simulink model "Vehicle_suspension"  (R2020b)
settings: Solver=VariableStepAuto  StartTime=0.0  StopTime=10.0  RelTol=1e-3
values from neighbouring files (symbols this model uses):
  Iyy = 2100.0    [data_dictionary.sldd]
  Mb = 1200.0    [data_dictionary.sldd]
undefined symbols (not defined in the file or in its folder): Cf, Cr, Kf, Kr, Lf, Lr, sigbuilder_block
settings Model: DataDictionary=data_dictionary.sldd  Creator=JAGRUTI SHINDE  LastModifiedBy=JAGRUTI SHINDE

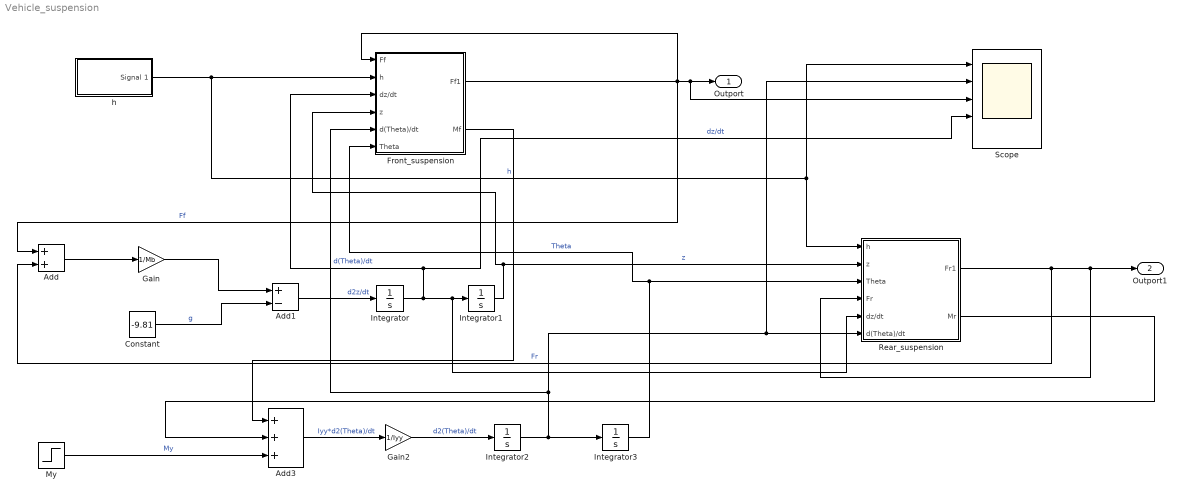
== system Vehicle_suspension ==
  Add : Sum
  Add1 : Sum  Inputs=+-
  Add3 : Sum  Inputs=+++
  Constant : Constant  Value=-9.81
  Front_suspension : Subsystem  InitFcn=|
      | Lf=0.9;
      | Kf=28000;
      | Cf=2500;
  Gain : Gain  Gain=1/Mb
  Gain2 : Gain  Gain=1/Iyy
  Integrator{,1..3} (4 alike) : Integrator
  My : Step  SampleTime=0
  Rear_suspension : Subsystem  InitFcn=|
      | Lr=1.2;
      | Kr=21000;
      | Cr=2000;
  Scope : Scope  NumInputPorts=5
  "h " : Subsystem  Tag=STV Subsys  LoadFcn=sigbuilder_block('load');  StartFcn=sigbuilder_block('start');  StopFcn=sigbuilder_block('stop');  ClipboardFcn=sigbuilder_block('clipboard');  mask(Sigbuilder block){tuvar=[0:10]}
      mask help: Simulink:masks:SigbuilderBlock_MD
      mask init:
      | if ~strcmp(get_param(bdroot(gcbh),'SimulationStatus'),'stopped') tuvar = sigbuilder_block('maskInit'); end
      settings: CopyFcn=sigbuilder_block('copy');  DeleteFcn=sigbuilder_block('delete');  ModelCloseFcn=sigbuilder_block('modelClose');  PreSaveFcn=sigbuilder_block('preSave');  PauseFcn=sigbuilder_block('pause');  ContinueFcn=sigbuilder_block('continue');  NameChangeFcn=sigbuilder_block('namechange');  OpenFcn=sigbuilder_block('open',[437.6 153 550.4 359.25 ]);  CloseFcn=sigbuilder_block('close');
      mask Display: plot(0, 0, 100, 100,[2, 2, 32, 32, 2], [68, 8, 8, 68, 68],[32, 2], [38, 38], [32, 19, 2],[53, 60, 44], [32, 17, 17, 2],[16, 16, 31, 31]);txt = getActiveGroup(gcbh);text(2, 100, txt,'verticalAlignment', 'top');
  Outport : Outport
  Outport1 : Outport  Port=2
  wires:
  Add/1 -> Gain/1
  Gain/1 -> Add1/1
  Constant/1 -> Add1/2  "g"
  Add1/1 -> Integrator/1  "d2z/dt"
  Integrator/1 -> Scope/4, Front_suspension/3(dz/dt), Rear_suspension/5(dz/dt), Integrator1/1  "dz/dt"
  My/1 -> Add3/3  "My"
  Add3/1 -> Gain2/1  "Iyy*d2(Theta)/dt"
  Gain2/1 -> Integrator2/1  "d2(Theta)/dt"
  Integrator2/1 -> Scope/2, Rear_suspension/6(d(Theta)/dt), Front_suspension/5(d(Theta)/dt), Integrator3/1  "d(Theta)/dt"
  Front_suspension/1(Ff1) -> Add/1, Scope/3, Outport/1, Front_suspension/1(Ff)  "Ff"
  "h "/1(Signal 1) -> Scope/1, Rear_suspension/1(h), Front_suspension/2(h)  "h"
  Integrator1/1 -> Front_suspension/4(z), Rear_suspension/2(z)  "z"
  Integrator3/1 -> Front_suspension/6(Theta), Rear_suspension/3(Theta)  "Theta"
  Front_suspension/2(Mf) -> Add3/1
  Rear_suspension/1(Fr1) -> Add/2, Rear_suspension/4(Fr), Outport1/1  "Fr"
  Rear_suspension/2(Mr) -> Add3/2

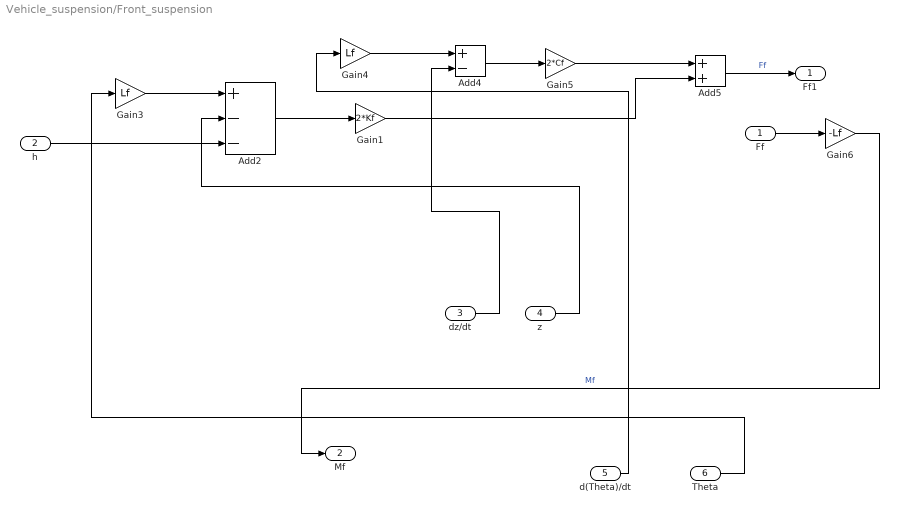
== system Vehicle_suspension/Front_suspension ==
  Ff : Inport
  h : Inport  Port=2
  dz/dt : Inport  Port=3
  z : Inport  Port=4
  d(Theta)/dt : Inport  Port=5
  Theta : Inport  Port=6
  Add2 : Sum  Inputs=+--
  Add4 : Sum  Inputs=+-
  Add5 : Sum
  Gain1 : Gain  Gain=2*Kf
  Gain3 : Gain  Gain=Lf
  Gain4 : Gain  Gain=Lf
  Gain5 : Gain  Gain=2*Cf
  Gain6 : Gain  Gain=-Lf
  Ff1 : Outport
  Mf : Outport  Port=2
  wires:
  d(Theta)/dt/1 -> Gain4/1
  Add4/1 -> Gain5/1
  z/1 -> Add2/2
  Gain4/1 -> Add4/1
  Gain3/1 -> Add2/1
  Gain5/1 -> Add5/1
  Gain1/1 -> Add5/2
  Add5/1 -> Ff1/1  "Ff"
  Theta/1 -> Gain3/1
  Add2/1 -> Gain1/1
  Gain6/1 -> Mf/1  "Mf"
  dz/dt/1 -> Add4/2
  h/1 -> Add2/3
  Ff/1 -> Gain6/1

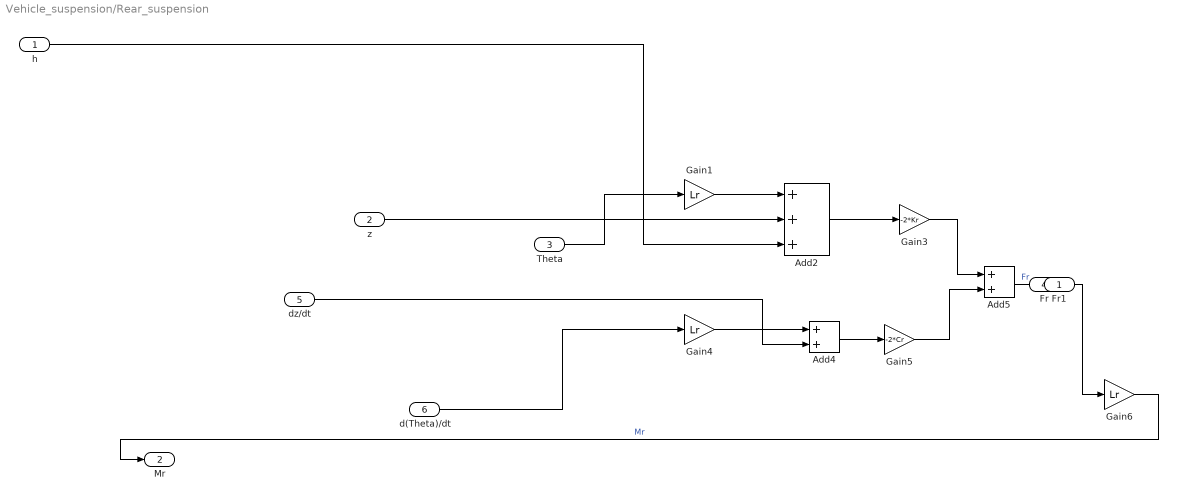
== system Vehicle_suspension/Rear_suspension ==
  h : Inport
  z : Inport  Port=2
  Theta : Inport  Port=3
  Fr : Inport  Port=4
  dz/dt : Inport  Port=5
  d(Theta)/dt : Inport  Port=6
  Add2 : Sum  Inputs=+++
  Add4 : Sum
  Add5 : Sum
  Gain1 : Gain  Gain=Lr
  Gain3 : Gain  Gain=-2*Kr
  Gain4 : Gain  Gain=Lr
  Gain5 : Gain  Gain=-2*Cr
  Gain6 : Gain  Gain=Lr
  Fr1 : Outport
  Mr : Outport  Port=2
  wires:
  z/1 -> Add2/2
  Gain3/1 -> Add5/1
  Add4/1 -> Gain5/1
  Gain1/1 -> Add2/1
  Fr/1 -> Gain6/1
  Add2/1 -> Gain3/1
  dz/dt/1 -> Add4/2
  Gain4/1 -> Add4/1
  Gain5/1 -> Add5/2
  d(Theta)/dt/1 -> Gain4/1
  Gain6/1 -> Mr/1  "Mr"
  Add5/1 -> Fr1/1  "Fr"
  h/1 -> Add2/3
  Theta/1 -> Gain1/1

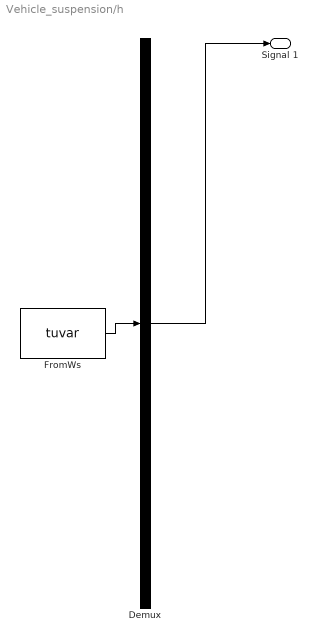
== system Vehicle_suspension/h  ==
  Demux : Demux  Tag=STV Demux  Outputs=1
      settings: DisplayOption=none
  FromWs : FromWorkspace  Tag=STV FromWs  VariableName=tuvar
      SigBuilderData=|
      | common.afterFinalStr = 'Extrapolate'
      | common.sampleTime = 0
      | dataSet.timeRange = [0 10]
      | dataSet.name = 'Group 1'
      | sbobj.Groups.Name = 'Group 1'
      | sbobj.Groups.Signals.Name = 'Signal 1'
      | sbobj.Groups.Signals.XData = [0 2 2 4 4 6 10]
      | sbobj.Groups.Signals.YData = [0 0 1 1 0 0 0]
  Signal 1 : Outport  Tag=STV Outport
  wires:
  Demux/1 -> Signal 1/1
  FromWs/1 -> Demux/1
